simulink model "mnpq"  (Simulink 3.00)
settings: Solver=ode45  SolverMode=SingleTasking  StartTime=0.0  StopTime=20  MaxStep=.010  RelTol=1e-3  AbsTol=1e-3
settings Model: TimeSaveName=t  SaveOutput=off

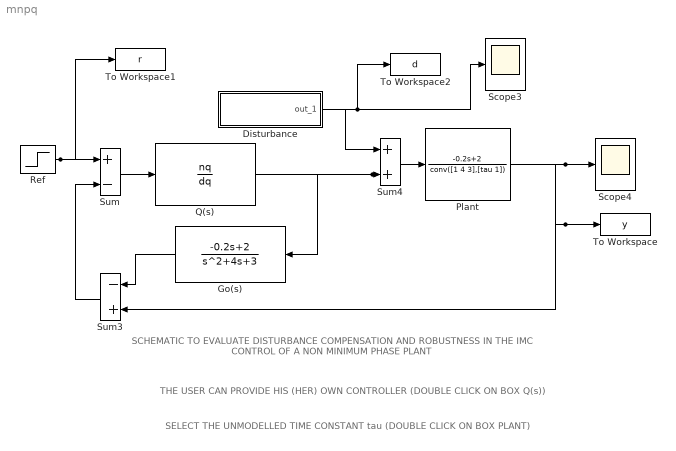
== system mnpq ==
  note: SCHEMATIC TO EVALUATE DISTURBANCE COMPENSATION AND  ROBUSTNESS
      | IN THE IMC CONTROL OF A NON MINIMUM PHASE PLANT
  note: THE USER CAN PROVIDE HIS (HER) OWN CONTROLLER (DOUBLE CLICK ON BOX Q(s))
  note: SELECT THE UNMODELLED TIME CONSTANT tau (DOUBLE CLICK ON BOX PLANT)
  Disturbance : Subsystem  mask(Input disturbance){@1=1, @2=0.5}
      mask prompts: @1 "Amplitude  of constant component:"; @2 "Amplitude  of varying component:"
      mask help: disturbance
      mask init:
      | Kc=@1;Kv=@2;
      mask Help: This block generates a signal with average value Kc and a varying component amplified by Kv
      mask Display: disp('Disturbance')
  Go(s) : TransferFcn  Orientation=left  Numerator=[-0.2 2]  Denominator=[1 4 3]
  Plant : TransferFcn  Numerator=[-0.2 2]  Denominator=conv([1 4 3],[tau 1])  mask(plant){@1=0}
      mask prompts: @1 "unmodelled time constant tau:"
      mask help: plant
      mask init:
      | tau=@1;
      mask Help: Plant with unmodelled dynamics. Enter tau=0 for perfect modelling
      mask Display: disp('PLANT')
  Q(s) : TransferFcn  Numerator=nq  Denominator=dq  mask(Q(s)){@1=[8 32 24], @2=[1 4 16]}
      mask prompts: @1 "numerator of Q(s):"; @2 "denominator of Q(s):"
      mask help: Q(s)
      mask init:
      | nq=@1;dq=@2;
      mask Display: disp('Q(s)')
  Ref : Step  Time=1  Before=0  After=1  SampleTime=0
  Scope3 : Scope
      settings: TickLabels=on  TimeRange=20.000000  YMin=-2.000000  YMax=2.000000  SaveToWorkspace=off  SaveName=ScopeData  DataFormat=Matrix
  Scope4 : Scope
      settings: TickLabels=on  TimeRange=20.000000  YMin=-2.000000  YMax=2.000000  SaveToWorkspace=off  SaveName=ScopeData  DataFormat=Matrix
  Sum : Sum  Inputs=+-  SaturateOnIntegerOverflow=on
  Sum3 : Sum  Orientation=left  Inputs=-+  SaturateOnIntegerOverflow=on
  Sum4 : Sum  Inputs=++  SaturateOnIntegerOverflow=on
  To Workspace : ToWorkspace  VariableName=y  SampleTime=0  SaveFormat=Matrix
      settings: Buffer=10000
  To Workspace1 : ToWorkspace  VariableName=r  SampleTime=0  SaveFormat=Matrix
      settings: Buffer=10000
  To Workspace2 : ToWorkspace  VariableName=d  SampleTime=0  SaveFormat=Matrix
      settings: Buffer=10000
  wires:
  Sum/1 -> Q(s)/1
  Go(s)/1 -> Sum3/1
  Sum3/1 -> Sum/2
  Q(s)/1 -> Sum4/2, Go(s)/1
  Plant/1 -> Scope4/1, Sum3/2, To Workspace/1
  Sum4/1 -> Plant/1
  Disturbance/1(out_1) -> Sum4/1, Scope3/1, To Workspace2/1
  Ref/1 -> Sum/1, To Workspace1/1

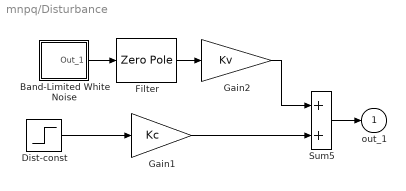
== system mnpq/Disturbance ==
  Band-Limited White Noise : Subsystem  mask(Continuous White Noise.){@1=[0.1], @2=0.1, @3=[23341]}
      mask prompts: @1 "Noise Power:"; @2 "Sample Time:"; @3 "Seed"
      mask help:
      | White noise for continuous (s-domain) systems.
      | Band-limited using zero-order-hold.
      mask init:
      | Cov = @1; Ts = @2; seed = @3; r = rand(1,12); r2 = [r(1),r;r,r(12)]; t =[1:13;1:13];
      mask Help: Implemented using white noise into Zero-Order Hold block. The seed and power can be vectors of the same length to produce a vector of white noise sources. For faster simulation, set sample time to the highest value possible but in accordance with the fastest dynamics of system.
      mask Display: plot(t(:),r2(:))
  Dist-const : Step  Time=0  Before=0  After=1  SampleTime=0
  Filter : ZeroPole  Zeros=z  Poles=p  Gain=k  mask(buttap){@1=4, @2=6}
      mask prompts: @1 "Cutoff frequency (rad/sec)"; @2 "Order"
      mask help:
      | Analog Butterworth low pass filter.
      |
      | (Requires Signal Processing Toolbox)
      mask init:
      | [z,p,k]=buttap(@2); z=@1*z; p=@1*p; k=real(prod(-p)); [num,den]=zp2tf(z,p,k); w=logspace(log10(@1/10),log10(10*@1),20); h=freqs(num,den,w);
      mask Help: Butterworth low pass filter using MATLAB's butter command.
      mask Display: plot(20*log10(w),20*log10(abs(h)))
  Gain1 : Gain  Gain=Kc  SaturateOnIntegerOverflow=on
  Gain2 : Gain  Gain=Kv  SaturateOnIntegerOverflow=on
  Sum5 : Sum  Inputs=++  SaturateOnIntegerOverflow=on
  out_1 : Outport  Port=1  InitialOutput=0
  wires:
  Gain2/1 -> Sum5/1
  Filter/1 -> Gain2/1
  Gain1/1 -> Sum5/2
  Band-Limited White Noise/1(Out_1) -> Filter/1
  Sum5/1 -> out_1/1
  Dist-const/1 -> Gain1/1

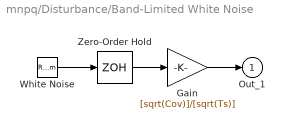
== system mnpq/Disturbance/Band-Limited White Noise ==
  Gain : Gain  Gain=[sqrt(Cov)]/[sqrt(Ts)]  SaturateOnIntegerOverflow=on
  White Noise : RandomNumber  Mean=0  Variance=1  Seed=seed  SampleTime=0
  Zero-Order Hold : ZeroOrderHold  SampleTime=Ts
  Out_1 : Outport  Port=1  InitialOutput=0
  wires:
  White Noise/1 -> Zero-Order Hold/1
  Gain/1 -> Out_1/1
  Zero-Order Hold/1 -> Gain/1
